simulink model "CSI_0313_4DC"  (R2018a)
settings: Solver=FixedStepDiscrete  StartTime=0.0  StopTime=Tstop  FixedStep=Tdelt  MaxStep=1e-4  RelTol=1e-3
values from neighbouring files (symbols this model uses):
  C = 12e-6    (= 1.2e-05)    [Inputparameter.m]
  Cdc = 4.76*10^-3    (= 0.00476)    [Inputparameter.m]
  Cemc = 1.5e-6    (= 1.5e-06)    [Inputparameter.m]
  fanalog = 7000    [Run.m]
  fKIUdc = 6    [Run.m]
  fKPUdc = 0.4    [Run.m]
  fTs = Update/18000    (= 0.000111111111111)    [Run.m]
  K120 = 0.0    (= 0)    [Run.m]
  K21 = 0.0    (= 0)    [Run.m]
  K5 = 0.0    (= 0)    [Run.m]
  K7 = 0.0    (= 0)    [Run.m]
  Kipll = 1.0    (= 1)    [Run.m]
  klmt = 0.3    [Run.m]
  Kpll = 20.0    (= 20)    [Run.m]
  Lgrid = 7.717e-4*10    (= 0.007717)    [Run.m]
  Lline = 60e-6    (= 6e-05)    [Inputparameter.m]
  Lpwm = 184.8e-6    (= 0.0001848)    [Inputparameter.m]
  mode = 1    [Run.m]
  Nsw = 18000/fbase    [Run.m]
  Qbpf = 1.0    (= 1)    [Run.m]
  Rc = 10e-3    (= 0.01)    [Inputparameter.m]
  Remc = 1e-3    (= 0.001)    [Inputparameter.m]
  Rgrid = 2*pi*fbase*Lgrid/XR    [Run.m]
  Rline = 4.95e-3    (= 0.00495)    [Inputparameter.m]
  Rpre = 2.2    [Inputparameter.m]
  Rpwm = 6.2e-3    (= 0.0062)    [Inputparameter.m]
  Tdelt = (fTs)/(200*Update)    (= 2.77777777778e-07)    [Run.m]
  Tdt = 1.27e-6    (= 1.27e-06)    [Run.m]
  tstart = 0.2    [Run.m]
  Tvstep = 1.5    [Run.m]
  Update = 2    [Run.m]
  Vbase = 400*sqrt(2/3)    [Inputparameter.m]
undefined symbols (not defined in the file or in its folder): sigbuilder_block
libraries: powerlib x412
(part 6 of 13)

== system CSI_0313_4DC/AIP1/Subsystem7/BPF  ==
  Vriz : Inport
  Freq : Inport  Port=2
  Demux1 : Demux  Outputs=3
  IIR_BPF_Re1 : MATLAB Function  TreatAsAtomicUnit=on  mask{fQ=Qbpf, fTs=fTs, iMode=IIR2 used as BPF in SOGI}
      mask prompts: fQ "Quality factor"; fTs "Sample time [s]"; iMode "Modes of 2nd-order transfer function"
  IIR_BPF_Re2 : MATLAB Function  TreatAsAtomicUnit=on  mask{fQ=Qbpf, fTs=fTs, iMode=IIR2 used as BPF in SOGI}
      mask prompts: fQ "Quality factor"; fTs "Sample time [s]"; iMode "Modes of 2nd-order transfer function"
  IIR_BPF_Re3 : MATLAB Function  TreatAsAtomicUnit=on  mask{fQ=Qbpf, fTs=fTs, iMode=IIR2 used as BPF in SOGI}
      mask prompts: fQ "Quality factor"; fTs "Sample time [s]"; iMode "Modes of 2nd-order transfer function"
  Mux1 : Mux  Inputs=3
  VpccBPF : Outport  VectorParamsAs1DForOutWhenUnconnected=on
  wires:
  Demux1/1 -> IIR_BPF_Re1/1(u)
  Mux1/1 -> VpccBPF/1
  Freq/1 -> IIR_BPF_Re3/2(fn), IIR_BPF_Re2/2(fn), IIR_BPF_Re1/2(fn)
  IIR_BPF_Re2/1(y) -> Mux1/2
  Demux1/2 -> IIR_BPF_Re2/1(u)
  Vriz/1 -> Demux1/1
  IIR_BPF_Re1/1(y) -> Mux1/1
  Demux1/3 -> IIR_BPF_Re3/1(u)
  IIR_BPF_Re3/1(y) -> Mux1/3

== system CSI_0313_4DC/AIP1/Subsystem7/Pos Compensation1 ==
  Vdc : Inport
  wt : Inport  Port=2
  Constant3 : Constant  Value=0  SampleTime=-1
  DQ0_To_RIZ : MATLAB Function  TreatAsAtomicUnit=on  mask{iAxis=orient in A-axis}
      mask prompts: iAxis "Orient Axis Choice"
  Gain2 : Gain  Gain=1/Vbase
  Gain3 : Gain  Gain=1/Vbase
  Gain4 : Gain  Gain=-1
  Ground : Ground
  Mux : Mux  Inputs=3
  PI Ctrl2 : MATLAB Function  TreatAsAtomicUnit=on  mask{fKP=fKPUdc, fKI=fKIUdc, fMinLmt=-klmt*Vbase, fMaxLmt=klmt*Vbase, fTs=fTs}
      mask prompts: fKP "Proportional Gain"; fKI "Integral Coefficient"; fMinLmt "Minimum Limitation"; fMaxLmt "Maximum Limitation"; fTs "Sampling time [s]"
      mask help: Proportional Resonant Controller
  RIZ_To_ABC : MATLAB Function  TreatAsAtomicUnit=on
  RIZ_To_DQ0 : MATLAB Function  TreatAsAtomicUnit=on  mask{iAxis=orient in A-axis}
      mask prompts: iAxis "Orient Axis Choice"
  Scope : Scope
  Scope1 : Scope
  Scope2 : Scope
  Scope6 : Scope  NumInputPorts=2
  Step : Step  Time=Tvstep  Before=650  After=700
  Sum1 : Sum  Inputs=|-+
  VabcFBPU : Outport
  wires:
  [Vdc] -> Sum1/2, Scope6/2
  PI Ctrl2/1(y) -> [VdRef]
  Sum1/1 -> PI Ctrl2/1(err)
  Vdc/1 -> [Vdc]
  [VabcFB] -> Scope1/1, Gain2/1
  [VdRef] -> Scope/1
  Ground/1 -> Mux/3
  Mux/1 -> DQ0_To_RIZ/1(DQ0)
  wt/1 -> RIZ_To_DQ0/2(wt), DQ0_To_RIZ/2(wt)
  RIZ_To_ABC/1(ABC) -> [VabcFB]
  DQ0_To_RIZ/1(RIZ) -> RIZ_To_DQ0/1(RIZ), RIZ_To_ABC/1(RIZ)
  Gain2/1 -> VabcFBPU/1
  Step/1 -> Scope6/1, Sum1/1
  RIZ_To_DQ0/1(DQ0) -> Gain3/1
  Gain3/1 -> Scope2/1
  [VdRef] -> Mux/2, Gain4/1
  Constant3/1 -> Mux/1

== system CSI_0313_4DC/AIP1/Subsystem7/Subsystem5 ==
  Vabc : Inport
  Vdc : Inport  Port=2
  3rd Injection1 : MATLAB Function  TreatAsAtomicUnit=on  mask{mode=mode}
      mask prompts: mode "Three wire/four wire"
  Vmod : Outport  VectorParamsAs1DForOutWhenUnconnected=on
  wires:
  Vabc/1 -> 3rd Injection1/1(Vabc)
  3rd Injection1/1(Mod) -> Vmod/1
  Vdc/1 -> 3rd Injection1/2(Vdc)

== system CSI_0313_4DC/AIP10/Subsystem5/PLL ==
  Vabc : Inport
  ABC_To_RIZ : MATLAB Function  TreatAsAtomicUnit=on
  Constant : Constant  Value=2*pi*fFqBase  SampleTime=-1
  Constant1 : Constant  Value=2*pi
  Delay1 : Delay  DelayLength=1
  Delay2 : Delay  DelayLength=1
  Demux3 : Demux  Outputs=3
  Gain : Gain  Gain=1/(2*pi)
  Integral : MATLAB Function  TreatAsAtomicUnit=on  mask{fGain=1.0, fTs=fTs}
      mask prompts: fGain "Gain Value"; fTs "Sampling time [s]"
      mask help: Proportional Resonant Controller
  Math Function : Math  Operator=mod  SaturateOnIntegerOverflow=on
  PI Ctrl : MATLAB Function  TreatAsAtomicUnit=on  mask{fKP=fKPPLL, fKI=fKIPLL, fMinLmt=fDltMin, fMaxLmt=fDltMax, fTs=fTs}
      mask prompts: fKP "Proportional Gain"; fKI "Integral Coefficient"; fMinLmt "Minimum Limitation"; fMaxLmt "Maximum Limitation"; fTs "Sampling time [s]"
      mask help: Proportional Resonant Controller
  "Pos&Neg seq extract in subsystem " : Subsystem  mask{fQ=1.0, fTs=fTs}
      mask prompts: fQ "Quality Factor"; fTs "Sample Time"
  RIZ_To_DQ0 : MATLAB Function  TreatAsAtomicUnit=on  mask{iAxis=orient in A-axis}
      mask prompts: iAxis "Orient Axis Choice"
  Scope : Scope
  Sum : Sum  Inputs=++|
  Terminator : Terminator
  Terminator1 : Terminator
  f : Outport  VectorParamsAs1DForOutWhenUnconnected=on
  wt : Outport  Port=2  VectorParamsAs1DForOutWhenUnconnected=on
  VdPos : Outport  Port=3  VectorParamsAs1DForOutWhenUnconnected=on
  wires:
  Delay1/1 -> "Pos&Neg seq extract in subsystem "/2(ffc)
  "Pos&Neg seq extract in subsystem "/3(chk) -> [chk]
  [f] -> Delay1/1
  Demux3/3 -> Terminator1/1
  "Pos&Neg seq extract in subsystem "/2(RizNeg) -> Terminator/1
  "Pos&Neg seq extract in subsystem "/1(RizPos) -> VdPos/1, [VrizPos]
  [Vriz] -> "Pos&Neg seq extract in subsystem "/1(RIZ)
  RIZ_To_DQ0/1(DQ0) -> Scope/1, [Vdq0Pos]
  [w] -> Gain/1
  [w] -> Integral/1(u)
  Gain/1 -> [f]
  Demux3/2 -> [VqPos]
  Demux3/1 -> [VdPos]
  [Vdq0Pos] -> Demux3/1
  PI Ctrl/1(y) -> Sum/2
  Sum/1 -> [w]
  [VrizPos] -> RIZ_To_DQ0/1(RIZ)
  Constant/1 -> Sum/1
  Vabc/1 -> [Vabc]
  Integral/1(y) -> Math Function/1
  Constant1/1 -> Math Function/2
  Math Function/1 -> [wt]
  [VqPos] -> PI Ctrl/1(err)
  [f] -> f/1
  [wt] -> Delay2/1
  Delay2/1 -> RIZ_To_DQ0/2(wt)
  [Vabc] -> ABC_To_RIZ/1(ABC)
  ABC_To_RIZ/1(RIZ) -> [Vriz]
  [wt] -> wt/1

== system CSI_0313_4DC/AIP10/Subsystem7/BPF  ==
  Vriz : Inport
  Freq : Inport  Port=2
  Demux1 : Demux  Outputs=3
  IIR_BPF_Re1 : MATLAB Function  TreatAsAtomicUnit=on  mask{fQ=Qbpf, fTs=fTs, iMode=IIR2 used as BPF in SOGI}
      mask prompts: fQ "Quality factor"; fTs "Sample time [s]"; iMode "Modes of 2nd-order transfer function"
  IIR_BPF_Re2 : MATLAB Function  TreatAsAtomicUnit=on  mask{fQ=Qbpf, fTs=fTs, iMode=IIR2 used as BPF in SOGI}
      mask prompts: fQ "Quality factor"; fTs "Sample time [s]"; iMode "Modes of 2nd-order transfer function"
  IIR_BPF_Re3 : MATLAB Function  TreatAsAtomicUnit=on  mask{fQ=Qbpf, fTs=fTs, iMode=IIR2 used as BPF in SOGI}
      mask prompts: fQ "Quality factor"; fTs "Sample time [s]"; iMode "Modes of 2nd-order transfer function"
  Mux1 : Mux  Inputs=3
  VpccBPF : Outport  VectorParamsAs1DForOutWhenUnconnected=on
  wires:
  Demux1/1 -> IIR_BPF_Re1/1(u)
  Mux1/1 -> VpccBPF/1
  Freq/1 -> IIR_BPF_Re3/2(fn), IIR_BPF_Re2/2(fn), IIR_BPF_Re1/2(fn)
  IIR_BPF_Re2/1(y) -> Mux1/2
  Demux1/2 -> IIR_BPF_Re2/1(u)
  Vriz/1 -> Demux1/1
  IIR_BPF_Re1/1(y) -> Mux1/1
  Demux1/3 -> IIR_BPF_Re3/1(u)
  IIR_BPF_Re3/1(y) -> Mux1/3

== system CSI_0313_4DC/AIP10/Subsystem7/Pos Compensation1 ==
  Vdc : Inport
  wt : Inport  Port=2
  Constant3 : Constant  Value=0  SampleTime=-1
  DQ0_To_RIZ : MATLAB Function  TreatAsAtomicUnit=on  mask{iAxis=orient in A-axis}
      mask prompts: iAxis "Orient Axis Choice"
  Gain2 : Gain  Gain=1/Vbase
  Gain3 : Gain  Gain=1/Vbase
  Gain4 : Gain  Gain=-1
  Ground : Ground
  Mux : Mux  Inputs=3
  PI Ctrl2 : MATLAB Function  TreatAsAtomicUnit=on  mask{fKP=fKPUdc, fKI=fKIUdc, fMinLmt=-klmt*Vbase, fMaxLmt=klmt*Vbase, fTs=fTs}
      mask prompts: fKP "Proportional Gain"; fKI "Integral Coefficient"; fMinLmt "Minimum Limitation"; fMaxLmt "Maximum Limitation"; fTs "Sampling time [s]"
      mask help: Proportional Resonant Controller
  RIZ_To_ABC : MATLAB Function  TreatAsAtomicUnit=on
  RIZ_To_DQ0 : MATLAB Function  TreatAsAtomicUnit=on  mask{iAxis=orient in A-axis}
      mask prompts: iAxis "Orient Axis Choice"
  Scope : Scope
  Scope1 : Scope
  Scope2 : Scope
  Scope6 : Scope  NumInputPorts=2
  Step : Step  Time=Tvstep  Before=650  After=700
  Sum1 : Sum  Inputs=|-+
  VabcFBPU : Outport
  wires:
  [Vdc] -> Sum1/2, Scope6/2
  PI Ctrl2/1(y) -> [VdRef]
  Sum1/1 -> PI Ctrl2/1(err)
  Vdc/1 -> [Vdc]
  [VabcFB] -> Scope1/1, Gain2/1
  [VdRef] -> Scope/1
  Ground/1 -> Mux/3
  Mux/1 -> DQ0_To_RIZ/1(DQ0)
  wt/1 -> RIZ_To_DQ0/2(wt), DQ0_To_RIZ/2(wt)
  RIZ_To_ABC/1(ABC) -> [VabcFB]
  DQ0_To_RIZ/1(RIZ) -> RIZ_To_DQ0/1(RIZ), RIZ_To_ABC/1(RIZ)
  Gain2/1 -> VabcFBPU/1
  Step/1 -> Scope6/1, Sum1/1
  RIZ_To_DQ0/1(DQ0) -> Gain3/1
  Gain3/1 -> Scope2/1
  [VdRef] -> Mux/2, Gain4/1
  Constant3/1 -> Mux/1

== system CSI_0313_4DC/AIP10/Subsystem7/Subsystem5 ==
  Vabc : Inport
  Vdc : Inport  Port=2
  3rd Injection1 : MATLAB Function  TreatAsAtomicUnit=on  mask{mode=mode}
      mask prompts: mode "Three wire/four wire"
  Vmod : Outport  VectorParamsAs1DForOutWhenUnconnected=on
  wires:
  Vabc/1 -> 3rd Injection1/1(Vabc)
  3rd Injection1/1(Mod) -> Vmod/1
  Vdc/1 -> 3rd Injection1/2(Vdc)

== system CSI_0313_4DC/AIP2/Subsystem5/PLL ==
  Vabc : Inport
  ABC_To_RIZ : MATLAB Function  TreatAsAtomicUnit=on
  Constant : Constant  Value=2*pi*fFqBase  SampleTime=-1
  Constant1 : Constant  Value=2*pi
  Delay1 : Delay  DelayLength=1
  Delay2 : Delay  DelayLength=1
  Demux3 : Demux  Outputs=3
  Gain : Gain  Gain=1/(2*pi)
  Integral : MATLAB Function  TreatAsAtomicUnit=on  mask{fGain=1.0, fTs=fTs}
      mask prompts: fGain "Gain Value"; fTs "Sampling time [s]"
      mask help: Proportional Resonant Controller
  Math Function : Math  Operator=mod  SaturateOnIntegerOverflow=on
  PI Ctrl : MATLAB Function  TreatAsAtomicUnit=on  mask{fKP=fKPPLL, fKI=fKIPLL, fMinLmt=fDltMin, fMaxLmt=fDltMax, fTs=fTs}
      mask prompts: fKP "Proportional Gain"; fKI "Integral Coefficient"; fMinLmt "Minimum Limitation"; fMaxLmt "Maximum Limitation"; fTs "Sampling time [s]"
      mask help: Proportional Resonant Controller
  "Pos&Neg seq extract in subsystem " : Subsystem  mask{fQ=1.0, fTs=fTs}
      mask prompts: fQ "Quality Factor"; fTs "Sample Time"
  RIZ_To_DQ0 : MATLAB Function  TreatAsAtomicUnit=on  mask{iAxis=orient in A-axis}
      mask prompts: iAxis "Orient Axis Choice"
  Scope : Scope
  Sum : Sum  Inputs=++|
  Terminator : Terminator
  Terminator1 : Terminator
  f : Outport  VectorParamsAs1DForOutWhenUnconnected=on
  wt : Outport  Port=2  VectorParamsAs1DForOutWhenUnconnected=on
  VdPos : Outport  Port=3  VectorParamsAs1DForOutWhenUnconnected=on
  wires:
  [wt] -> wt/1
  ABC_To_RIZ/1(RIZ) -> [Vriz]
  [Vabc] -> ABC_To_RIZ/1(ABC)
  Delay2/1 -> RIZ_To_DQ0/2(wt)
  [wt] -> Delay2/1
  [f] -> f/1
  [VqPos] -> PI Ctrl/1(err)
  Math Function/1 -> [wt]
  Constant1/1 -> Math Function/2
  Integral/1(y) -> Math Function/1
  Vabc/1 -> [Vabc]
  Constant/1 -> Sum/1
  [VrizPos] -> RIZ_To_DQ0/1(RIZ)
  Sum/1 -> [w]
  PI Ctrl/1(y) -> Sum/2
  [Vdq0Pos] -> Demux3/1
  Demux3/1 -> [VdPos]
  Demux3/2 -> [VqPos]
  Gain/1 -> [f]
  [w] -> Integral/1(u)
  [w] -> Gain/1
  RIZ_To_DQ0/1(DQ0) -> [Vdq0Pos], Scope/1
  [Vriz] -> "Pos&Neg seq extract in subsystem "/1(RIZ)
  "Pos&Neg seq extract in subsystem "/1(RizPos) -> [VrizPos], VdPos/1
  "Pos&Neg seq extract in subsystem "/2(RizNeg) -> Terminator/1
  Demux3/3 -> Terminator1/1
  [f] -> Delay1/1
  "Pos&Neg seq extract in subsystem "/3(chk) -> [chk]
  Delay1/1 -> "Pos&Neg seq extract in subsystem "/2(ffc)

== system CSI_0313_4DC/AIP2/Subsystem7/BPF  ==
  Vriz : Inport
  Freq : Inport  Port=2
  Demux1 : Demux  Outputs=3
  IIR_BPF_Re1 : MATLAB Function  TreatAsAtomicUnit=on  mask{fQ=Qbpf, fTs=fTs, iMode=IIR2 used as BPF in SOGI}
      mask prompts: fQ "Quality factor"; fTs "Sample time [s]"; iMode "Modes of 2nd-order transfer function"
  IIR_BPF_Re2 : MATLAB Function  TreatAsAtomicUnit=on  mask{fQ=Qbpf, fTs=fTs, iMode=IIR2 used as BPF in SOGI}
      mask prompts: fQ "Quality factor"; fTs "Sample time [s]"; iMode "Modes of 2nd-order transfer function"
  IIR_BPF_Re3 : MATLAB Function  TreatAsAtomicUnit=on  mask{fQ=Qbpf, fTs=fTs, iMode=IIR2 used as BPF in SOGI}
      mask prompts: fQ "Quality factor"; fTs "Sample time [s]"; iMode "Modes of 2nd-order transfer function"
  Mux1 : Mux  Inputs=3
  VpccBPF : Outport  VectorParamsAs1DForOutWhenUnconnected=on
  wires:
  IIR_BPF_Re3/1(y) -> Mux1/3
  Demux1/3 -> IIR_BPF_Re3/1(u)
  IIR_BPF_Re1/1(y) -> Mux1/1
  Vriz/1 -> Demux1/1
  Demux1/2 -> IIR_BPF_Re2/1(u)
  IIR_BPF_Re2/1(y) -> Mux1/2
  Freq/1 -> IIR_BPF_Re1/2(fn), IIR_BPF_Re2/2(fn), IIR_BPF_Re3/2(fn)
  Mux1/1 -> VpccBPF/1
  Demux1/1 -> IIR_BPF_Re1/1(u)

== system CSI_0313_4DC/AIP2/Subsystem7/Pos Compensation1 ==
  Vdc : Inport
  wt : Inport  Port=2
  Constant3 : Constant  Value=0  SampleTime=-1
  DQ0_To_RIZ : MATLAB Function  TreatAsAtomicUnit=on  mask{iAxis=orient in A-axis}
      mask prompts: iAxis "Orient Axis Choice"
  Gain2 : Gain  Gain=1/Vbase
  Gain3 : Gain  Gain=1/Vbase
  Gain4 : Gain  Gain=-1
  Ground : Ground
  Mux : Mux  Inputs=3
  PI Ctrl2 : MATLAB Function  TreatAsAtomicUnit=on  mask{fKP=fKPUdc, fKI=fKIUdc, fMinLmt=-klmt*Vbase, fMaxLmt=klmt*Vbase, fTs=fTs}
      mask prompts: fKP "Proportional Gain"; fKI "Integral Coefficient"; fMinLmt "Minimum Limitation"; fMaxLmt "Maximum Limitation"; fTs "Sampling time [s]"
      mask help: Proportional Resonant Controller
  RIZ_To_ABC : MATLAB Function  TreatAsAtomicUnit=on
  RIZ_To_DQ0 : MATLAB Function  TreatAsAtomicUnit=on  mask{iAxis=orient in A-axis}
      mask prompts: iAxis "Orient Axis Choice"
  Scope : Scope
  Scope1 : Scope
  Scope2 : Scope
  Scope6 : Scope  NumInputPorts=2
  Step : Step  Time=Tvstep  Before=650  After=700
  Sum1 : Sum  Inputs=|-+
  VabcFBPU : Outport
  wires:
  Constant3/1 -> Mux/1
  [VdRef] -> Gain4/1, Mux/2
  Gain3/1 -> Scope2/1
  RIZ_To_DQ0/1(DQ0) -> Gain3/1
  Step/1 -> Sum1/1, Scope6/1
  Gain2/1 -> VabcFBPU/1
  DQ0_To_RIZ/1(RIZ) -> RIZ_To_ABC/1(RIZ), RIZ_To_DQ0/1(RIZ)
  RIZ_To_ABC/1(ABC) -> [VabcFB]
  wt/1 -> DQ0_To_RIZ/2(wt), RIZ_To_DQ0/2(wt)
  Mux/1 -> DQ0_To_RIZ/1(DQ0)
  Ground/1 -> Mux/3
  [VdRef] -> Scope/1
  [VabcFB] -> Gain2/1, Scope1/1
  Vdc/1 -> [Vdc]
  Sum1/1 -> PI Ctrl2/1(err)
  PI Ctrl2/1(y) -> [VdRef]
  [Vdc] -> Scope6/2, Sum1/2

== system CSI_0313_4DC/AIP2/Subsystem7/Subsystem5 ==
  Vabc : Inport
  Vdc : Inport  Port=2
  3rd Injection1 : MATLAB Function  TreatAsAtomicUnit=on  mask{mode=mode}
      mask prompts: mode "Three wire/four wire"
  Vmod : Outport  VectorParamsAs1DForOutWhenUnconnected=on
  wires:
  Vdc/1 -> 3rd Injection1/2(Vdc)
  3rd Injection1/1(Mod) -> Vmod/1
  Vabc/1 -> 3rd Injection1/1(Vabc)

== system CSI_0313_4DC/AIP3/Subsystem5/PLL ==
  Vabc : Inport
  ABC_To_RIZ : MATLAB Function  TreatAsAtomicUnit=on
  Constant : Constant  Value=2*pi*fFqBase  SampleTime=-1
  Constant1 : Constant  Value=2*pi
  Delay1 : Delay  DelayLength=1
  Delay2 : Delay  DelayLength=1
  Demux3 : Demux  Outputs=3
  Gain : Gain  Gain=1/(2*pi)
  Integral : MATLAB Function  TreatAsAtomicUnit=on  mask{fGain=1.0, fTs=fTs}
      mask prompts: fGain "Gain Value"; fTs "Sampling time [s]"
      mask help: Proportional Resonant Controller
  Math Function : Math  Operator=mod  SaturateOnIntegerOverflow=on
  PI Ctrl : MATLAB Function  TreatAsAtomicUnit=on  mask{fKP=fKPPLL, fKI=fKIPLL, fMinLmt=fDltMin, fMaxLmt=fDltMax, fTs=fTs}
      mask prompts: fKP "Proportional Gain"; fKI "Integral Coefficient"; fMinLmt "Minimum Limitation"; fMaxLmt "Maximum Limitation"; fTs "Sampling time [s]"
      mask help: Proportional Resonant Controller
  "Pos&Neg seq extract in subsystem " : Subsystem  mask{fQ=1.0, fTs=fTs}
      mask prompts: fQ "Quality Factor"; fTs "Sample Time"
  RIZ_To_DQ0 : MATLAB Function  TreatAsAtomicUnit=on  mask{iAxis=orient in A-axis}
      mask prompts: iAxis "Orient Axis Choice"
  Scope : Scope
  Sum : Sum  Inputs=++|
  Terminator : Terminator
  Terminator1 : Terminator
  f : Outport  VectorParamsAs1DForOutWhenUnconnected=on
  wt : Outport  Port=2  VectorParamsAs1DForOutWhenUnconnected=on
  VdPos : Outport  Port=3  VectorParamsAs1DForOutWhenUnconnected=on
  wires:
  Delay1/1 -> "Pos&Neg seq extract in subsystem "/2(ffc)
  "Pos&Neg seq extract in subsystem "/3(chk) -> [chk]
  [f] -> Delay1/1
  Demux3/3 -> Terminator1/1
  "Pos&Neg seq extract in subsystem "/2(RizNeg) -> Terminator/1
  "Pos&Neg seq extract in subsystem "/1(RizPos) -> VdPos/1, [VrizPos]
  [Vriz] -> "Pos&Neg seq extract in subsystem "/1(RIZ)
  RIZ_To_DQ0/1(DQ0) -> Scope/1, [Vdq0Pos]
  [w] -> Gain/1
  [w] -> Integral/1(u)
  Gain/1 -> [f]
  Demux3/2 -> [VqPos]
  Demux3/1 -> [VdPos]
  [Vdq0Pos] -> Demux3/1
  PI Ctrl/1(y) -> Sum/2
  Sum/1 -> [w]
  [VrizPos] -> RIZ_To_DQ0/1(RIZ)
  Constant/1 -> Sum/1
  Vabc/1 -> [Vabc]
  Integral/1(y) -> Math Function/1
  Constant1/1 -> Math Function/2
  Math Function/1 -> [wt]
  [VqPos] -> PI Ctrl/1(err)
  [f] -> f/1
  [wt] -> Delay2/1
  Delay2/1 -> RIZ_To_DQ0/2(wt)
  [Vabc] -> ABC_To_RIZ/1(ABC)
  ABC_To_RIZ/1(RIZ) -> [Vriz]
  [wt] -> wt/1

== system CSI_0313_4DC/AIP3/Subsystem7/BPF  ==
  Vriz : Inport
  Freq : Inport  Port=2
  Demux1 : Demux  Outputs=3
  IIR_BPF_Re1 : MATLAB Function  TreatAsAtomicUnit=on  mask{fQ=Qbpf, fTs=fTs, iMode=IIR2 used as BPF in SOGI}
      mask prompts: fQ "Quality factor"; fTs "Sample time [s]"; iMode "Modes of 2nd-order transfer function"
  IIR_BPF_Re2 : MATLAB Function  TreatAsAtomicUnit=on  mask{fQ=Qbpf, fTs=fTs, iMode=IIR2 used as BPF in SOGI}
      mask prompts: fQ "Quality factor"; fTs "Sample time [s]"; iMode "Modes of 2nd-order transfer function"
  IIR_BPF_Re3 : MATLAB Function  TreatAsAtomicUnit=on  mask{fQ=Qbpf, fTs=fTs, iMode=IIR2 used as BPF in SOGI}
      mask prompts: fQ "Quality factor"; fTs "Sample time [s]"; iMode "Modes of 2nd-order transfer function"
  Mux1 : Mux  Inputs=3
  VpccBPF : Outport  VectorParamsAs1DForOutWhenUnconnected=on
  wires:
  Demux1/1 -> IIR_BPF_Re1/1(u)
  Mux1/1 -> VpccBPF/1
  Freq/1 -> IIR_BPF_Re3/2(fn), IIR_BPF_Re2/2(fn), IIR_BPF_Re1/2(fn)
  IIR_BPF_Re2/1(y) -> Mux1/2
  Demux1/2 -> IIR_BPF_Re2/1(u)
  Vriz/1 -> Demux1/1
  IIR_BPF_Re1/1(y) -> Mux1/1
  Demux1/3 -> IIR_BPF_Re3/1(u)
  IIR_BPF_Re3/1(y) -> Mux1/3

== system CSI_0313_4DC/AIP3/Subsystem7/Pos Compensation1 ==
  Vdc : Inport
  wt : Inport  Port=2
  Constant3 : Constant  Value=0  SampleTime=-1
  DQ0_To_RIZ : MATLAB Function  TreatAsAtomicUnit=on  mask{iAxis=orient in A-axis}
      mask prompts: iAxis "Orient Axis Choice"
  Gain2 : Gain  Gain=1/Vbase
  Gain3 : Gain  Gain=1/Vbase
  Gain4 : Gain  Gain=-1
  Ground : Ground
  Mux : Mux  Inputs=3
  PI Ctrl2 : MATLAB Function  TreatAsAtomicUnit=on  mask{fKP=fKPUdc, fKI=fKIUdc, fMinLmt=-klmt*Vbase, fMaxLmt=klmt*Vbase, fTs=fTs}
      mask prompts: fKP "Proportional Gain"; fKI "Integral Coefficient"; fMinLmt "Minimum Limitation"; fMaxLmt "Maximum Limitation"; fTs "Sampling time [s]"
      mask help: Proportional Resonant Controller
  RIZ_To_ABC : MATLAB Function  TreatAsAtomicUnit=on
  RIZ_To_DQ0 : MATLAB Function  TreatAsAtomicUnit=on  mask{iAxis=orient in A-axis}
      mask prompts: iAxis "Orient Axis Choice"
  Scope : Scope
  Scope1 : Scope
  Scope2 : Scope
  Scope6 : Scope  NumInputPorts=2
  Step : Step  Time=Tvstep  Before=650  After=700
  Sum1 : Sum  Inputs=|-+
  VabcFBPU : Outport
  wires:
  [Vdc] -> Sum1/2, Scope6/2
  PI Ctrl2/1(y) -> [VdRef]
  Sum1/1 -> PI Ctrl2/1(err)
  Vdc/1 -> [Vdc]
  [VabcFB] -> Scope1/1, Gain2/1
  [VdRef] -> Scope/1
  Ground/1 -> Mux/3
  Mux/1 -> DQ0_To_RIZ/1(DQ0)
  wt/1 -> RIZ_To_DQ0/2(wt), DQ0_To_RIZ/2(wt)
  RIZ_To_ABC/1(ABC) -> [VabcFB]
  DQ0_To_RIZ/1(RIZ) -> RIZ_To_DQ0/1(RIZ), RIZ_To_ABC/1(RIZ)
  Gain2/1 -> VabcFBPU/1
  Step/1 -> Scope6/1, Sum1/1
  RIZ_To_DQ0/1(DQ0) -> Gain3/1
  Gain3/1 -> Scope2/1
  [VdRef] -> Mux/2, Gain4/1
  Constant3/1 -> Mux/1

== system CSI_0313_4DC/AIP3/Subsystem7/Subsystem5 ==
  Vabc : Inport
  Vdc : Inport  Port=2
  3rd Injection1 : MATLAB Function  TreatAsAtomicUnit=on  mask{mode=mode}
      mask prompts: mode "Three wire/four wire"
  Vmod : Outport  VectorParamsAs1DForOutWhenUnconnected=on
  wires:
  Vabc/1 -> 3rd Injection1/1(Vabc)
  3rd Injection1/1(Mod) -> Vmod/1
  Vdc/1 -> 3rd Injection1/2(Vdc)

== system CSI_0313_4DC/AIP4/Subsystem5/PLL ==
  Vabc : Inport
  ABC_To_RIZ : MATLAB Function  TreatAsAtomicUnit=on
  Constant : Constant  Value=2*pi*fFqBase  SampleTime=-1
  Constant1 : Constant  Value=2*pi
  Delay1 : Delay  DelayLength=1
  Delay2 : Delay  DelayLength=1
  Demux3 : Demux  Outputs=3
  Gain : Gain  Gain=1/(2*pi)
  Integral : MATLAB Function  TreatAsAtomicUnit=on  mask{fGain=1.0, fTs=fTs}
      mask prompts: fGain "Gain Value"; fTs "Sampling time [s]"
      mask help: Proportional Resonant Controller
  Math Function : Math  Operator=mod  SaturateOnIntegerOverflow=on
  PI Ctrl : MATLAB Function  TreatAsAtomicUnit=on  mask{fKP=fKPPLL, fKI=fKIPLL, fMinLmt=fDltMin, fMaxLmt=fDltMax, fTs=fTs}
      mask prompts: fKP "Proportional Gain"; fKI "Integral Coefficient"; fMinLmt "Minimum Limitation"; fMaxLmt "Maximum Limitation"; fTs "Sampling time [s]"
      mask help: Proportional Resonant Controller
  "Pos&Neg seq extract in subsystem " : Subsystem  mask{fQ=1.0, fTs=fTs}
      mask prompts: fQ "Quality Factor"; fTs "Sample Time"
  RIZ_To_DQ0 : MATLAB Function  TreatAsAtomicUnit=on  mask{iAxis=orient in A-axis}
      mask prompts: iAxis "Orient Axis Choice"
  Scope : Scope
  Sum : Sum  Inputs=++|
  Terminator : Terminator
  Terminator1 : Terminator
  f : Outport  VectorParamsAs1DForOutWhenUnconnected=on
  wt : Outport  Port=2  VectorParamsAs1DForOutWhenUnconnected=on
  VdPos : Outport  Port=3  VectorParamsAs1DForOutWhenUnconnected=on
  wires:
  [wt] -> wt/1
  ABC_To_RIZ/1(RIZ) -> [Vriz]
  [Vabc] -> ABC_To_RIZ/1(ABC)
  Delay2/1 -> RIZ_To_DQ0/2(wt)
  [wt] -> Delay2/1
  [f] -> f/1
  [VqPos] -> PI Ctrl/1(err)
  Math Function/1 -> [wt]
  Constant1/1 -> Math Function/2
  Integral/1(y) -> Math Function/1
  Vabc/1 -> [Vabc]
  Constant/1 -> Sum/1
  [VrizPos] -> RIZ_To_DQ0/1(RIZ)
  Sum/1 -> [w]
  PI Ctrl/1(y) -> Sum/2
  [Vdq0Pos] -> Demux3/1
  Demux3/1 -> [VdPos]
  Demux3/2 -> [VqPos]
  Gain/1 -> [f]
  [w] -> Integral/1(u)
  [w] -> Gain/1
  RIZ_To_DQ0/1(DQ0) -> [Vdq0Pos], Scope/1
  [Vriz] -> "Pos&Neg seq extract in subsystem "/1(RIZ)
  "Pos&Neg seq extract in subsystem "/1(RizPos) -> [VrizPos], VdPos/1
  "Pos&Neg seq extract in subsystem "/2(RizNeg) -> Terminator/1
  Demux3/3 -> Terminator1/1
  [f] -> Delay1/1
  "Pos&Neg seq extract in subsystem "/3(chk) -> [chk]
  Delay1/1 -> "Pos&Neg seq extract in subsystem "/2(ffc)

== system CSI_0313_4DC/AIP4/Subsystem7/BPF  ==
  Vriz : Inport
  Freq : Inport  Port=2
  Demux1 : Demux  Outputs=3
  IIR_BPF_Re1 : MATLAB Function  TreatAsAtomicUnit=on  mask{fQ=Qbpf, fTs=fTs, iMode=IIR2 used as BPF in SOGI}
      mask prompts: fQ "Quality factor"; fTs "Sample time [s]"; iMode "Modes of 2nd-order transfer function"
  IIR_BPF_Re2 : MATLAB Function  TreatAsAtomicUnit=on  mask{fQ=Qbpf, fTs=fTs, iMode=IIR2 used as BPF in SOGI}
      mask prompts: fQ "Quality factor"; fTs "Sample time [s]"; iMode "Modes of 2nd-order transfer function"
  IIR_BPF_Re3 : MATLAB Function  TreatAsAtomicUnit=on  mask{fQ=Qbpf, fTs=fTs, iMode=IIR2 used as BPF in SOGI}
      mask prompts: fQ "Quality factor"; fTs "Sample time [s]"; iMode "Modes of 2nd-order transfer function"
  Mux1 : Mux  Inputs=3
  VpccBPF : Outport  VectorParamsAs1DForOutWhenUnconnected=on
  wires:
  IIR_BPF_Re3/1(y) -> Mux1/3
  Demux1/3 -> IIR_BPF_Re3/1(u)
  IIR_BPF_Re1/1(y) -> Mux1/1
  Vriz/1 -> Demux1/1
  Demux1/2 -> IIR_BPF_Re2/1(u)
  IIR_BPF_Re2/1(y) -> Mux1/2
  Freq/1 -> IIR_BPF_Re1/2(fn), IIR_BPF_Re2/2(fn), IIR_BPF_Re3/2(fn)
  Mux1/1 -> VpccBPF/1
  Demux1/1 -> IIR_BPF_Re1/1(u)

== system CSI_0313_4DC/AIP4/Subsystem7/Pos Compensation1 ==
  Vdc : Inport
  wt : Inport  Port=2
  Constant3 : Constant  Value=0  SampleTime=-1
  DQ0_To_RIZ : MATLAB Function  TreatAsAtomicUnit=on  mask{iAxis=orient in A-axis}
      mask prompts: iAxis "Orient Axis Choice"
  Gain2 : Gain  Gain=1/Vbase
  Gain3 : Gain  Gain=1/Vbase
  Gain4 : Gain  Gain=-1
  Ground : Ground
  Mux : Mux  Inputs=3
  PI Ctrl2 : MATLAB Function  TreatAsAtomicUnit=on  mask{fKP=fKPUdc, fKI=fKIUdc, fMinLmt=-klmt*Vbase, fMaxLmt=klmt*Vbase, fTs=fTs}
      mask prompts: fKP "Proportional Gain"; fKI "Integral Coefficient"; fMinLmt "Minimum Limitation"; fMaxLmt "Maximum Limitation"; fTs "Sampling time [s]"
      mask help: Proportional Resonant Controller
  RIZ_To_ABC : MATLAB Function  TreatAsAtomicUnit=on
  RIZ_To_DQ0 : MATLAB Function  TreatAsAtomicUnit=on  mask{iAxis=orient in A-axis}
      mask prompts: iAxis "Orient Axis Choice"
  Scope : Scope
  Scope1 : Scope
  Scope2 : Scope
  Scope6 : Scope  NumInputPorts=2
  Step : Step  Time=Tvstep  Before=650  After=700
  Sum1 : Sum  Inputs=|-+
  VabcFBPU : Outport
  wires:
  Constant3/1 -> Mux/1
  [VdRef] -> Gain4/1, Mux/2
  Gain3/1 -> Scope2/1
  RIZ_To_DQ0/1(DQ0) -> Gain3/1
  Step/1 -> Sum1/1, Scope6/1
  Gain2/1 -> VabcFBPU/1
  DQ0_To_RIZ/1(RIZ) -> RIZ_To_ABC/1(RIZ), RIZ_To_DQ0/1(RIZ)
  RIZ_To_ABC/1(ABC) -> [VabcFB]
  wt/1 -> DQ0_To_RIZ/2(wt), RIZ_To_DQ0/2(wt)
  Mux/1 -> DQ0_To_RIZ/1(DQ0)
  Ground/1 -> Mux/3
  [VdRef] -> Scope/1
  [VabcFB] -> Gain2/1, Scope1/1
  Vdc/1 -> [Vdc]
  Sum1/1 -> PI Ctrl2/1(err)
  PI Ctrl2/1(y) -> [VdRef]
  [Vdc] -> Scope6/2, Sum1/2

== system CSI_0313_4DC/AIP4/Subsystem7/Subsystem5 ==
  Vabc : Inport
  Vdc : Inport  Port=2
  3rd Injection1 : MATLAB Function  TreatAsAtomicUnit=on  mask{mode=mode}
      mask prompts: mode "Three wire/four wire"
  Vmod : Outport  VectorParamsAs1DForOutWhenUnconnected=on
  wires:
  Vdc/1 -> 3rd Injection1/2(Vdc)
  3rd Injection1/1(Mod) -> Vmod/1
  Vabc/1 -> 3rd Injection1/1(Vabc)

== system CSI_0313_4DC/AIP5/Subsystem5/PLL ==
  Vabc : Inport
  ABC_To_RIZ : MATLAB Function  TreatAsAtomicUnit=on
  Constant : Constant  Value=2*pi*fFqBase  SampleTime=-1
  Constant1 : Constant  Value=2*pi
  Delay1 : Delay  DelayLength=1
  Delay2 : Delay  DelayLength=1
  Demux3 : Demux  Outputs=3
  Gain : Gain  Gain=1/(2*pi)
  Integral : MATLAB Function  TreatAsAtomicUnit=on  mask{fGain=1.0, fTs=fTs}
      mask prompts: fGain "Gain Value"; fTs "Sampling time [s]"
      mask help: Proportional Resonant Controller
  Math Function : Math  Operator=mod  SaturateOnIntegerOverflow=on
  PI Ctrl : MATLAB Function  TreatAsAtomicUnit=on  mask{fKP=fKPPLL, fKI=fKIPLL, fMinLmt=fDltMin, fMaxLmt=fDltMax, fTs=fTs}
      mask prompts: fKP "Proportional Gain"; fKI "Integral Coefficient"; fMinLmt "Minimum Limitation"; fMaxLmt "Maximum Limitation"; fTs "Sampling time [s]"
      mask help: Proportional Resonant Controller
  "Pos&Neg seq extract in subsystem " : Subsystem  mask{fQ=1.0, fTs=fTs}
      mask prompts: fQ "Quality Factor"; fTs "Sample Time"
  RIZ_To_DQ0 : MATLAB Function  TreatAsAtomicUnit=on  mask{iAxis=orient in A-axis}
      mask prompts: iAxis "Orient Axis Choice"
  Scope : Scope
  Sum : Sum  Inputs=++|
  Terminator : Terminator
  Terminator1 : Terminator
  f : Outport  VectorParamsAs1DForOutWhenUnconnected=on
  wt : Outport  Port=2  VectorParamsAs1DForOutWhenUnconnected=on
  VdPos : Outport  Port=3  VectorParamsAs1DForOutWhenUnconnected=on
  wires:
  Delay1/1 -> "Pos&Neg seq extract in subsystem "/2(ffc)
  "Pos&Neg seq extract in subsystem "/3(chk) -> [chk]
  [f] -> Delay1/1
  Demux3/3 -> Terminator1/1
  "Pos&Neg seq extract in subsystem "/2(RizNeg) -> Terminator/1
  "Pos&Neg seq extract in subsystem "/1(RizPos) -> VdPos/1, [VrizPos]
  [Vriz] -> "Pos&Neg seq extract in subsystem "/1(RIZ)
  RIZ_To_DQ0/1(DQ0) -> Scope/1, [Vdq0Pos]
  [w] -> Gain/1
  [w] -> Integral/1(u)
  Gain/1 -> [f]
  Demux3/2 -> [VqPos]
  Demux3/1 -> [VdPos]
  [Vdq0Pos] -> Demux3/1
  PI Ctrl/1(y) -> Sum/2
  Sum/1 -> [w]
  [VrizPos] -> RIZ_To_DQ0/1(RIZ)
  Constant/1 -> Sum/1
  Vabc/1 -> [Vabc]
  Integral/1(y) -> Math Function/1
  Constant1/1 -> Math Function/2
  Math Function/1 -> [wt]
  [VqPos] -> PI Ctrl/1(err)
  [f] -> f/1
  [wt] -> Delay2/1
  Delay2/1 -> RIZ_To_DQ0/2(wt)
  [Vabc] -> ABC_To_RIZ/1(ABC)
  ABC_To_RIZ/1(RIZ) -> [Vriz]
  [wt] -> wt/1

== system CSI_0313_4DC/AIP5/Subsystem7/BPF  ==
  Vriz : Inport
  Freq : Inport  Port=2
  Demux1 : Demux  Outputs=3
  IIR_BPF_Re1 : MATLAB Function  TreatAsAtomicUnit=on  mask{fQ=Qbpf, fTs=fTs, iMode=IIR2 used as BPF in SOGI}
      mask prompts: fQ "Quality factor"; fTs "Sample time [s]"; iMode "Modes of 2nd-order transfer function"
  IIR_BPF_Re2 : MATLAB Function  TreatAsAtomicUnit=on  mask{fQ=Qbpf, fTs=fTs, iMode=IIR2 used as BPF in SOGI}
      mask prompts: fQ "Quality factor"; fTs "Sample time [s]"; iMode "Modes of 2nd-order transfer function"
  IIR_BPF_Re3 : MATLAB Function  TreatAsAtomicUnit=on  mask{fQ=Qbpf, fTs=fTs, iMode=IIR2 used as BPF in SOGI}
      mask prompts: fQ "Quality factor"; fTs "Sample time [s]"; iMode "Modes of 2nd-order transfer function"
  Mux1 : Mux  Inputs=3
  VpccBPF : Outport  VectorParamsAs1DForOutWhenUnconnected=on
  wires:
  Demux1/1 -> IIR_BPF_Re1/1(u)
  Mux1/1 -> VpccBPF/1
  Freq/1 -> IIR_BPF_Re3/2(fn), IIR_BPF_Re2/2(fn), IIR_BPF_Re1/2(fn)
  IIR_BPF_Re2/1(y) -> Mux1/2
  Demux1/2 -> IIR_BPF_Re2/1(u)
  Vriz/1 -> Demux1/1
  IIR_BPF_Re1/1(y) -> Mux1/1
  Demux1/3 -> IIR_BPF_Re3/1(u)
  IIR_BPF_Re3/1(y) -> Mux1/3

== system CSI_0313_4DC/AIP5/Subsystem7/Pos Compensation1 ==
  Vdc : Inport
  wt : Inport  Port=2
  Constant3 : Constant  Value=0  SampleTime=-1
  DQ0_To_RIZ : MATLAB Function  TreatAsAtomicUnit=on  mask{iAxis=orient in A-axis}
      mask prompts: iAxis "Orient Axis Choice"
  Gain2 : Gain  Gain=1/Vbase
  Gain3 : Gain  Gain=1/Vbase
  Gain4 : Gain  Gain=-1
  Ground : Ground
  Mux : Mux  Inputs=3
  PI Ctrl2 : MATLAB Function  TreatAsAtomicUnit=on  mask{fKP=fKPUdc, fKI=fKIUdc, fMinLmt=-klmt*Vbase, fMaxLmt=klmt*Vbase, fTs=fTs}
      mask prompts: fKP "Proportional Gain"; fKI "Integral Coefficient"; fMinLmt "Minimum Limitation"; fMaxLmt "Maximum Limitation"; fTs "Sampling time [s]"
      mask help: Proportional Resonant Controller
  RIZ_To_ABC : MATLAB Function  TreatAsAtomicUnit=on
  RIZ_To_DQ0 : MATLAB Function  TreatAsAtomicUnit=on  mask{iAxis=orient in A-axis}
      mask prompts: iAxis "Orient Axis Choice"
  Scope : Scope
  Scope1 : Scope
  Scope2 : Scope
  Scope6 : Scope  NumInputPorts=2
  Step : Step  Time=Tvstep  Before=650  After=700
  Sum1 : Sum  Inputs=|-+
  VabcFBPU : Outport
  wires:
  [Vdc] -> Sum1/2, Scope6/2
  PI Ctrl2/1(y) -> [VdRef]
  Sum1/1 -> PI Ctrl2/1(err)
  Vdc/1 -> [Vdc]
  [VabcFB] -> Scope1/1, Gain2/1
  [VdRef] -> Scope/1
  Ground/1 -> Mux/3
  Mux/1 -> DQ0_To_RIZ/1(DQ0)
  wt/1 -> RIZ_To_DQ0/2(wt), DQ0_To_RIZ/2(wt)
  RIZ_To_ABC/1(ABC) -> [VabcFB]
  DQ0_To_RIZ/1(RIZ) -> RIZ_To_DQ0/1(RIZ), RIZ_To_ABC/1(RIZ)
  Gain2/1 -> VabcFBPU/1
  Step/1 -> Scope6/1, Sum1/1
  RIZ_To_DQ0/1(DQ0) -> Gain3/1
  Gain3/1 -> Scope2/1
  [VdRef] -> Mux/2, Gain4/1
  Constant3/1 -> Mux/1

== system CSI_0313_4DC/AIP5/Subsystem7/Subsystem5 ==
  Vabc : Inport
  Vdc : Inport  Port=2
  3rd Injection1 : MATLAB Function  TreatAsAtomicUnit=on  mask{mode=mode}
      mask prompts: mode "Three wire/four wire"
  Vmod : Outport  VectorParamsAs1DForOutWhenUnconnected=on
  wires:
  Vabc/1 -> 3rd Injection1/1(Vabc)
  3rd Injection1/1(Mod) -> Vmod/1
  Vdc/1 -> 3rd Injection1/2(Vdc)

== system CSI_0313_4DC/AIP6/Subsystem5/PLL ==
  Vabc : Inport
  ABC_To_RIZ : MATLAB Function  TreatAsAtomicUnit=on
  Constant : Constant  Value=2*pi*fFqBase  SampleTime=-1
  Constant1 : Constant  Value=2*pi
  Delay1 : Delay  DelayLength=1
  Delay2 : Delay  DelayLength=1
  Demux3 : Demux  Outputs=3
  Gain : Gain  Gain=1/(2*pi)
  Integral : MATLAB Function  TreatAsAtomicUnit=on  mask{fGain=1.0, fTs=fTs}
      mask prompts: fGain "Gain Value"; fTs "Sampling time [s]"
      mask help: Proportional Resonant Controller
  Math Function : Math  Operator=mod  SaturateOnIntegerOverflow=on
  PI Ctrl : MATLAB Function  TreatAsAtomicUnit=on  mask{fKP=fKPPLL, fKI=fKIPLL, fMinLmt=fDltMin, fMaxLmt=fDltMax, fTs=fTs}
      mask prompts: fKP "Proportional Gain"; fKI "Integral Coefficient"; fMinLmt "Minimum Limitation"; fMaxLmt "Maximum Limitation"; fTs "Sampling time [s]"
      mask help: Proportional Resonant Controller
  "Pos&Neg seq extract in subsystem " : Subsystem  mask{fQ=1.0, fTs=fTs}
      mask prompts: fQ "Quality Factor"; fTs "Sample Time"
  RIZ_To_DQ0 : MATLAB Function  TreatAsAtomicUnit=on  mask{iAxis=orient in A-axis}
      mask prompts: iAxis "Orient Axis Choice"
  Scope : Scope
  Sum : Sum  Inputs=++|
  Terminator : Terminator
  Terminator1 : Terminator
  f : Outport  VectorParamsAs1DForOutWhenUnconnected=on
  wt : Outport  Port=2  VectorParamsAs1DForOutWhenUnconnected=on
  VdPos : Outport  Port=3  VectorParamsAs1DForOutWhenUnconnected=on
  wires:
  Delay1/1 -> "Pos&Neg seq extract in subsystem "/2(ffc)
  "Pos&Neg seq extract in subsystem "/3(chk) -> [chk]
  [f] -> Delay1/1
  Demux3/3 -> Terminator1/1
  "Pos&Neg seq extract in subsystem "/2(RizNeg) -> Terminator/1
  "Pos&Neg seq extract in subsystem "/1(RizPos) -> VdPos/1, [VrizPos]
  [Vriz] -> "Pos&Neg seq extract in subsystem "/1(RIZ)
  RIZ_To_DQ0/1(DQ0) -> Scope/1, [Vdq0Pos]
  [w] -> Gain/1
  [w] -> Integral/1(u)
  Gain/1 -> [f]
  Demux3/2 -> [VqPos]
  Demux3/1 -> [VdPos]
  [Vdq0Pos] -> Demux3/1
  PI Ctrl/1(y) -> Sum/2
  Sum/1 -> [w]
  [VrizPos] -> RIZ_To_DQ0/1(RIZ)
  Constant/1 -> Sum/1
  Vabc/1 -> [Vabc]
  Integral/1(y) -> Math Function/1
  Constant1/1 -> Math Function/2
  Math Function/1 -> [wt]
  [VqPos] -> PI Ctrl/1(err)
  [f] -> f/1
  [wt] -> Delay2/1
  Delay2/1 -> RIZ_To_DQ0/2(wt)
  [Vabc] -> ABC_To_RIZ/1(ABC)
  ABC_To_RIZ/1(RIZ) -> [Vriz]
  [wt] -> wt/1

== system CSI_0313_4DC/AIP6/Subsystem7/BPF  ==
  Vriz : Inport
  Freq : Inport  Port=2
  Demux1 : Demux  Outputs=3
  IIR_BPF_Re1 : MATLAB Function  TreatAsAtomicUnit=on  mask{fQ=Qbpf, fTs=fTs, iMode=IIR2 used as BPF in SOGI}
      mask prompts: fQ "Quality factor"; fTs "Sample time [s]"; iMode "Modes of 2nd-order transfer function"
  IIR_BPF_Re2 : MATLAB Function  TreatAsAtomicUnit=on  mask{fQ=Qbpf, fTs=fTs, iMode=IIR2 used as BPF in SOGI}
      mask prompts: fQ "Quality factor"; fTs "Sample time [s]"; iMode "Modes of 2nd-order transfer function"
  IIR_BPF_Re3 : MATLAB Function  TreatAsAtomicUnit=on  mask{fQ=Qbpf, fTs=fTs, iMode=IIR2 used as BPF in SOGI}
      mask prompts: fQ "Quality factor"; fTs "Sample time [s]"; iMode "Modes of 2nd-order transfer function"
  Mux1 : Mux  Inputs=3
  VpccBPF : Outport  VectorParamsAs1DForOutWhenUnconnected=on
  wires:
  Demux1/1 -> IIR_BPF_Re1/1(u)
  Mux1/1 -> VpccBPF/1
  Freq/1 -> IIR_BPF_Re3/2(fn), IIR_BPF_Re2/2(fn), IIR_BPF_Re1/2(fn)
  IIR_BPF_Re2/1(y) -> Mux1/2
  Demux1/2 -> IIR_BPF_Re2/1(u)
  Vriz/1 -> Demux1/1
  IIR_BPF_Re1/1(y) -> Mux1/1
  Demux1/3 -> IIR_BPF_Re3/1(u)
  IIR_BPF_Re3/1(y) -> Mux1/3

== system CSI_0313_4DC/AIP6/Subsystem7/Pos Compensation1 ==
  Vdc : Inport
  wt : Inport  Port=2
  Constant3 : Constant  Value=0  SampleTime=-1
  DQ0_To_RIZ : MATLAB Function  TreatAsAtomicUnit=on  mask{iAxis=orient in A-axis}
      mask prompts: iAxis "Orient Axis Choice"
  Gain2 : Gain  Gain=1/Vbase
  Gain3 : Gain  Gain=1/Vbase
  Gain4 : Gain  Gain=-1
  Ground : Ground
  Mux : Mux  Inputs=3
  PI Ctrl2 : MATLAB Function  TreatAsAtomicUnit=on  mask{fKP=fKPUdc, fKI=fKIUdc, fMinLmt=-klmt*Vbase, fMaxLmt=klmt*Vbase, fTs=fTs}
      mask prompts: fKP "Proportional Gain"; fKI "Integral Coefficient"; fMinLmt "Minimum Limitation"; fMaxLmt "Maximum Limitation"; fTs "Sampling time [s]"
      mask help: Proportional Resonant Controller
  RIZ_To_ABC : MATLAB Function  TreatAsAtomicUnit=on
  RIZ_To_DQ0 : MATLAB Function  TreatAsAtomicUnit=on  mask{iAxis=orient in A-axis}
      mask prompts: iAxis "Orient Axis Choice"
  Scope : Scope
  Scope1 : Scope
  Scope2 : Scope
  Scope6 : Scope  NumInputPorts=2
  Step : Step  Time=Tvstep  Before=650  After=700
  Sum1 : Sum  Inputs=|-+
  VabcFBPU : Outport
  wires:
  [Vdc] -> Sum1/2, Scope6/2
  PI Ctrl2/1(y) -> [VdRef]
  Sum1/1 -> PI Ctrl2/1(err)
  Vdc/1 -> [Vdc]
  [VabcFB] -> Scope1/1, Gain2/1
  [VdRef] -> Scope/1
  Ground/1 -> Mux/3
  Mux/1 -> DQ0_To_RIZ/1(DQ0)
  wt/1 -> RIZ_To_DQ0/2(wt), DQ0_To_RIZ/2(wt)
  RIZ_To_ABC/1(ABC) -> [VabcFB]
  DQ0_To_RIZ/1(RIZ) -> RIZ_To_DQ0/1(RIZ), RIZ_To_ABC/1(RIZ)
  Gain2/1 -> VabcFBPU/1
  Step/1 -> Scope6/1, Sum1/1
  RIZ_To_DQ0/1(DQ0) -> Gain3/1
  Gain3/1 -> Scope2/1
  [VdRef] -> Mux/2, Gain4/1
  Constant3/1 -> Mux/1

== system CSI_0313_4DC/AIP6/Subsystem7/Subsystem5 ==
  Vabc : Inport
  Vdc : Inport  Port=2
  3rd Injection1 : MATLAB Function  TreatAsAtomicUnit=on  mask{mode=mode}
      mask prompts: mode "Three wire/four wire"
  Vmod : Outport  VectorParamsAs1DForOutWhenUnconnected=on
  wires:
  Vabc/1 -> 3rd Injection1/1(Vabc)
  3rd Injection1/1(Mod) -> Vmod/1
  Vdc/1 -> 3rd Injection1/2(Vdc)

== system CSI_0313_4DC/AIP7/Subsystem5/PLL ==
  Vabc : Inport
  ABC_To_RIZ : MATLAB Function  TreatAsAtomicUnit=on
  Constant : Constant  Value=2*pi*fFqBase  SampleTime=-1
  Constant1 : Constant  Value=2*pi
  Delay1 : Delay  DelayLength=1
  Delay2 : Delay  DelayLength=1
  Demux3 : Demux  Outputs=3
  Gain : Gain  Gain=1/(2*pi)
  Integral : MATLAB Function  TreatAsAtomicUnit=on  mask{fGain=1.0, fTs=fTs}
      mask prompts: fGain "Gain Value"; fTs "Sampling time [s]"
      mask help: Proportional Resonant Controller
  Math Function : Math  Operator=mod  SaturateOnIntegerOverflow=on
  PI Ctrl : MATLAB Function  TreatAsAtomicUnit=on  mask{fKP=fKPPLL, fKI=fKIPLL, fMinLmt=fDltMin, fMaxLmt=fDltMax, fTs=fTs}
      mask prompts: fKP "Proportional Gain"; fKI "Integral Coefficient"; fMinLmt "Minimum Limitation"; fMaxLmt "Maximum Limitation"; fTs "Sampling time [s]"
      mask help: Proportional Resonant Controller
  "Pos&Neg seq extract in subsystem " : Subsystem  mask{fQ=1.0, fTs=fTs}
      mask prompts: fQ "Quality Factor"; fTs "Sample Time"
  RIZ_To_DQ0 : MATLAB Function  TreatAsAtomicUnit=on  mask{iAxis=orient in A-axis}
      mask prompts: iAxis "Orient Axis Choice"
  Scope : Scope
  Sum : Sum  Inputs=++|
  Terminator : Terminator
  Terminator1 : Terminator
  f : Outport  VectorParamsAs1DForOutWhenUnconnected=on
  wt : Outport  Port=2  VectorParamsAs1DForOutWhenUnconnected=on
  VdPos : Outport  Port=3  VectorParamsAs1DForOutWhenUnconnected=on
  wires:
  [wt] -> wt/1
  ABC_To_RIZ/1(RIZ) -> [Vriz]
  [Vabc] -> ABC_To_RIZ/1(ABC)
  Delay2/1 -> RIZ_To_DQ0/2(wt)
  [wt] -> Delay2/1
  [f] -> f/1
  [VqPos] -> PI Ctrl/1(err)
  Math Function/1 -> [wt]
  Constant1/1 -> Math Function/2
  Integral/1(y) -> Math Function/1
  Vabc/1 -> [Vabc]
  Constant/1 -> Sum/1
  [VrizPos] -> RIZ_To_DQ0/1(RIZ)
  Sum/1 -> [w]
  PI Ctrl/1(y) -> Sum/2
  [Vdq0Pos] -> Demux3/1
  Demux3/1 -> [VdPos]
  Demux3/2 -> [VqPos]
  Gain/1 -> [f]
  [w] -> Integral/1(u)
  [w] -> Gain/1
  RIZ_To_DQ0/1(DQ0) -> [Vdq0Pos], Scope/1
  [Vriz] -> "Pos&Neg seq extract in subsystem "/1(RIZ)
  "Pos&Neg seq extract in subsystem "/1(RizPos) -> [VrizPos], VdPos/1
  "Pos&Neg seq extract in subsystem "/2(RizNeg) -> Terminator/1
  Demux3/3 -> Terminator1/1
  [f] -> Delay1/1
  "Pos&Neg seq extract in subsystem "/3(chk) -> [chk]
  Delay1/1 -> "Pos&Neg seq extract in subsystem "/2(ffc)

== system CSI_0313_4DC/AIP7/Subsystem7/BPF  ==
  Vriz : Inport
  Freq : Inport  Port=2
  Demux1 : Demux  Outputs=3
  IIR_BPF_Re1 : MATLAB Function  TreatAsAtomicUnit=on  mask{fQ=Qbpf, fTs=fTs, iMode=IIR2 used as BPF in SOGI}
      mask prompts: fQ "Quality factor"; fTs "Sample time [s]"; iMode "Modes of 2nd-order transfer function"
  IIR_BPF_Re2 : MATLAB Function  TreatAsAtomicUnit=on  mask{fQ=Qbpf, fTs=fTs, iMode=IIR2 used as BPF in SOGI}
      mask prompts: fQ "Quality factor"; fTs "Sample time [s]"; iMode "Modes of 2nd-order transfer function"
  IIR_BPF_Re3 : MATLAB Function  TreatAsAtomicUnit=on  mask{fQ=Qbpf, fTs=fTs, iMode=IIR2 used as BPF in SOGI}
      mask prompts: fQ "Quality factor"; fTs "Sample time [s]"; iMode "Modes of 2nd-order transfer function"
  Mux1 : Mux  Inputs=3
  VpccBPF : Outport  VectorParamsAs1DForOutWhenUnconnected=on
  wires:
  IIR_BPF_Re3/1(y) -> Mux1/3
  Demux1/3 -> IIR_BPF_Re3/1(u)
  IIR_BPF_Re1/1(y) -> Mux1/1
  Vriz/1 -> Demux1/1
  Demux1/2 -> IIR_BPF_Re2/1(u)
  IIR_BPF_Re2/1(y) -> Mux1/2
  Freq/1 -> IIR_BPF_Re1/2(fn), IIR_BPF_Re2/2(fn), IIR_BPF_Re3/2(fn)
  Mux1/1 -> VpccBPF/1
  Demux1/1 -> IIR_BPF_Re1/1(u)

== system CSI_0313_4DC/AIP7/Subsystem7/Pos Compensation1 ==
  Vdc : Inport
  wt : Inport  Port=2
  Constant3 : Constant  Value=0  SampleTime=-1
  DQ0_To_RIZ : MATLAB Function  TreatAsAtomicUnit=on  mask{iAxis=orient in A-axis}
      mask prompts: iAxis "Orient Axis Choice"
  Gain2 : Gain  Gain=1/Vbase
  Gain3 : Gain  Gain=1/Vbase
  Gain4 : Gain  Gain=-1
  Ground : Ground
  Mux : Mux  Inputs=3
  PI Ctrl2 : MATLAB Function  TreatAsAtomicUnit=on  mask{fKP=fKPUdc, fKI=fKIUdc, fMinLmt=-klmt*Vbase, fMaxLmt=klmt*Vbase, fTs=fTs}
      mask prompts: fKP "Proportional Gain"; fKI "Integral Coefficient"; fMinLmt "Minimum Limitation"; fMaxLmt "Maximum Limitation"; fTs "Sampling time [s]"
      mask help: Proportional Resonant Controller
  RIZ_To_ABC : MATLAB Function  TreatAsAtomicUnit=on
  RIZ_To_DQ0 : MATLAB Function  TreatAsAtomicUnit=on  mask{iAxis=orient in A-axis}
      mask prompts: iAxis "Orient Axis Choice"
  Scope : Scope
  Scope1 : Scope
  Scope2 : Scope
  Scope6 : Scope  NumInputPorts=2
  Step : Step  Time=Tvstep  Before=650  After=700
  Sum1 : Sum  Inputs=|-+
  VabcFBPU : Outport
  wires:
  Constant3/1 -> Mux/1
  [VdRef] -> Gain4/1, Mux/2
  Gain3/1 -> Scope2/1
  RIZ_To_DQ0/1(DQ0) -> Gain3/1
  Step/1 -> Sum1/1, Scope6/1
  Gain2/1 -> VabcFBPU/1
  DQ0_To_RIZ/1(RIZ) -> RIZ_To_ABC/1(RIZ), RIZ_To_DQ0/1(RIZ)
  RIZ_To_ABC/1(ABC) -> [VabcFB]
  wt/1 -> DQ0_To_RIZ/2(wt), RIZ_To_DQ0/2(wt)
  Mux/1 -> DQ0_To_RIZ/1(DQ0)
  Ground/1 -> Mux/3
  [VdRef] -> Scope/1
  [VabcFB] -> Gain2/1, Scope1/1
  Vdc/1 -> [Vdc]
  Sum1/1 -> PI Ctrl2/1(err)
  PI Ctrl2/1(y) -> [VdRef]
  [Vdc] -> Scope6/2, Sum1/2

== system CSI_0313_4DC/AIP7/Subsystem7/Subsystem5 ==
  Vabc : Inport
  Vdc : Inport  Port=2
  3rd Injection1 : MATLAB Function  TreatAsAtomicUnit=on  mask{mode=mode}
      mask prompts: mode "Three wire/four wire"
  Vmod : Outport  VectorParamsAs1DForOutWhenUnconnected=on
  wires:
  Vdc/1 -> 3rd Injection1/2(Vdc)
  3rd Injection1/1(Mod) -> Vmod/1
  Vabc/1 -> 3rd Injection1/1(Vabc)

== system CSI_0313_4DC/AIP8/Subsystem5/PLL ==
  Vabc : Inport
  ABC_To_RIZ : MATLAB Function  TreatAsAtomicUnit=on
  Constant : Constant  Value=2*pi*fFqBase  SampleTime=-1
  Constant1 : Constant  Value=2*pi
  Delay1 : Delay  DelayLength=1
  Delay2 : Delay  DelayLength=1
  Demux3 : Demux  Outputs=3
  Gain : Gain  Gain=1/(2*pi)
  Integral : MATLAB Function  TreatAsAtomicUnit=on  mask{fGain=1.0, fTs=fTs}
      mask prompts: fGain "Gain Value"; fTs "Sampling time [s]"
      mask help: Proportional Resonant Controller
  Math Function : Math  Operator=mod  SaturateOnIntegerOverflow=on
  PI Ctrl : MATLAB Function  TreatAsAtomicUnit=on  mask{fKP=fKPPLL, fKI=fKIPLL, fMinLmt=fDltMin, fMaxLmt=fDltMax, fTs=fTs}
      mask prompts: fKP "Proportional Gain"; fKI "Integral Coefficient"; fMinLmt "Minimum Limitation"; fMaxLmt "Maximum Limitation"; fTs "Sampling time [s]"
      mask help: Proportional Resonant Controller
  "Pos&Neg seq extract in subsystem " : Subsystem  mask{fQ=1.0, fTs=fTs}
      mask prompts: fQ "Quality Factor"; fTs "Sample Time"
  RIZ_To_DQ0 : MATLAB Function  TreatAsAtomicUnit=on  mask{iAxis=orient in A-axis}
      mask prompts: iAxis "Orient Axis Choice"
  Scope : Scope
  Sum : Sum  Inputs=++|
  Terminator : Terminator
  Terminator1 : Terminator
  f : Outport  VectorParamsAs1DForOutWhenUnconnected=on
  wt : Outport  Port=2  VectorParamsAs1DForOutWhenUnconnected=on
  VdPos : Outport  Port=3  VectorParamsAs1DForOutWhenUnconnected=on
  wires:
  Delay1/1 -> "Pos&Neg seq extract in subsystem "/2(ffc)
  "Pos&Neg seq extract in subsystem "/3(chk) -> [chk]
  [f] -> Delay1/1
  Demux3/3 -> Terminator1/1
  "Pos&Neg seq extract in subsystem "/2(RizNeg) -> Terminator/1
  "Pos&Neg seq extract in subsystem "/1(RizPos) -> VdPos/1, [VrizPos]
  [Vriz] -> "Pos&Neg seq extract in subsystem "/1(RIZ)
  RIZ_To_DQ0/1(DQ0) -> Scope/1, [Vdq0Pos]
  [w] -> Gain/1
  [w] -> Integral/1(u)
  Gain/1 -> [f]
  Demux3/2 -> [VqPos]
  Demux3/1 -> [VdPos]
  [Vdq0Pos] -> Demux3/1
  PI Ctrl/1(y) -> Sum/2
  Sum/1 -> [w]
  [VrizPos] -> RIZ_To_DQ0/1(RIZ)
  Constant/1 -> Sum/1
  Vabc/1 -> [Vabc]
  Integral/1(y) -> Math Function/1
  Constant1/1 -> Math Function/2
  Math Function/1 -> [wt]
  [VqPos] -> PI Ctrl/1(err)
  [f] -> f/1
  [wt] -> Delay2/1
  Delay2/1 -> RIZ_To_DQ0/2(wt)
  [Vabc] -> ABC_To_RIZ/1(ABC)
  ABC_To_RIZ/1(RIZ) -> [Vriz]
  [wt] -> wt/1

== system CSI_0313_4DC/AIP8/Subsystem7/BPF  ==
  Vriz : Inport
  Freq : Inport  Port=2
  Demux1 : Demux  Outputs=3
  IIR_BPF_Re1 : MATLAB Function  TreatAsAtomicUnit=on  mask{fQ=Qbpf, fTs=fTs, iMode=IIR2 used as BPF in SOGI}
      mask prompts: fQ "Quality factor"; fTs "Sample time [s]"; iMode "Modes of 2nd-order transfer function"
  IIR_BPF_Re2 : MATLAB Function  TreatAsAtomicUnit=on  mask{fQ=Qbpf, fTs=fTs, iMode=IIR2 used as BPF in SOGI}
      mask prompts: fQ "Quality factor"; fTs "Sample time [s]"; iMode "Modes of 2nd-order transfer function"
  IIR_BPF_Re3 : MATLAB Function  TreatAsAtomicUnit=on  mask{fQ=Qbpf, fTs=fTs, iMode=IIR2 used as BPF in SOGI}
      mask prompts: fQ "Quality factor"; fTs "Sample time [s]"; iMode "Modes of 2nd-order transfer function"
  Mux1 : Mux  Inputs=3
  VpccBPF : Outport  VectorParamsAs1DForOutWhenUnconnected=on
  wires:
  Demux1/1 -> IIR_BPF_Re1/1(u)
  Mux1/1 -> VpccBPF/1
  Freq/1 -> IIR_BPF_Re3/2(fn), IIR_BPF_Re2/2(fn), IIR_BPF_Re1/2(fn)
  IIR_BPF_Re2/1(y) -> Mux1/2
  Demux1/2 -> IIR_BPF_Re2/1(u)
  Vriz/1 -> Demux1/1
  IIR_BPF_Re1/1(y) -> Mux1/1
  Demux1/3 -> IIR_BPF_Re3/1(u)
  IIR_BPF_Re3/1(y) -> Mux1/3

== system CSI_0313_4DC/AIP8/Subsystem7/Pos Compensation1 ==
  Vdc : Inport
  wt : Inport  Port=2
  Constant3 : Constant  Value=0  SampleTime=-1
  DQ0_To_RIZ : MATLAB Function  TreatAsAtomicUnit=on  mask{iAxis=orient in A-axis}
      mask prompts: iAxis "Orient Axis Choice"
  Gain2 : Gain  Gain=1/Vbase
  Gain3 : Gain  Gain=1/Vbase
  Gain4 : Gain  Gain=-1
  Ground : Ground
  Mux : Mux  Inputs=3
  PI Ctrl2 : MATLAB Function  TreatAsAtomicUnit=on  mask{fKP=fKPUdc, fKI=fKIUdc, fMinLmt=-klmt*Vbase, fMaxLmt=klmt*Vbase, fTs=fTs}
      mask prompts: fKP "Proportional Gain"; fKI "Integral Coefficient"; fMinLmt "Minimum Limitation"; fMaxLmt "Maximum Limitation"; fTs "Sampling time [s]"
      mask help: Proportional Resonant Controller
  RIZ_To_ABC : MATLAB Function  TreatAsAtomicUnit=on
  RIZ_To_DQ0 : MATLAB Function  TreatAsAtomicUnit=on  mask{iAxis=orient in A-axis}
      mask prompts: iAxis "Orient Axis Choice"
  Scope : Scope
  Scope1 : Scope
  Scope2 : Scope
  Scope6 : Scope  NumInputPorts=2
  Step : Step  Time=Tvstep  Before=650  After=700
  Sum1 : Sum  Inputs=|-+
  VabcFBPU : Outport
  wires:
  [Vdc] -> Sum1/2, Scope6/2
  PI Ctrl2/1(y) -> [VdRef]
  Sum1/1 -> PI Ctrl2/1(err)
  Vdc/1 -> [Vdc]
  [VabcFB] -> Scope1/1, Gain2/1
  [VdRef] -> Scope/1
  Ground/1 -> Mux/3
  Mux/1 -> DQ0_To_RIZ/1(DQ0)
  wt/1 -> RIZ_To_DQ0/2(wt), DQ0_To_RIZ/2(wt)
  RIZ_To_ABC/1(ABC) -> [VabcFB]
  DQ0_To_RIZ/1(RIZ) -> RIZ_To_DQ0/1(RIZ), RIZ_To_ABC/1(RIZ)
  Gain2/1 -> VabcFBPU/1
  Step/1 -> Scope6/1, Sum1/1
  RIZ_To_DQ0/1(DQ0) -> Gain3/1
  Gain3/1 -> Scope2/1
  [VdRef] -> Mux/2, Gain4/1
  Constant3/1 -> Mux/1

== system CSI_0313_4DC/AIP8/Subsystem7/Subsystem5 ==
  Vabc : Inport
  Vdc : Inport  Port=2
  3rd Injection1 : MATLAB Function  TreatAsAtomicUnit=on  mask{mode=mode}
      mask prompts: mode "Three wire/four wire"
  Vmod : Outport  VectorParamsAs1DForOutWhenUnconnected=on
  wires:
  Vabc/1 -> 3rd Injection1/1(Vabc)
  3rd Injection1/1(Mod) -> Vmod/1
  Vdc/1 -> 3rd Injection1/2(Vdc)
